simulink model "controllers"  (R2022a)
settings: Solver=FixedStepDiscrete  StartTime=0.0  StopTime=30  FixedStep=1  RelTol=1e-3  EnableMultiTasking=on
settings Model: ExtModeTrigDuration=2  Creator=Amin  LastModifiedBy=Parsa Noori
settings SolverCC: AlgebraicLoopSolver=TrustRegion
settings OptimizationCC: DefaultParameterBehavior=Inlined  UseDivisionForNetSlopeComputation=on  GainParamInheritBuiltInType=on  UseFloatMulNetSlope=on  InlineInvariantSignals=on  PassReuseOutputArgsAs=Individual arguments  ZeroExternalMemoryAtStartup=off  ZeroInternalMemoryAtStartup=off  NoFixptDivByZeroProtection=on  EfficientFloat2IntCast=on  LifeSpan=1  MaxStackSize=64  OptimizeBlockOrder=speed  DifferentSizesBufferReuse=on  EfficientTunableParamExpr=on
settings DebuggingCC: ParameterTunabilityLossMsg=error  UnconnectedInputMsg=warning  UnconnectedOutputMsg=warning  UnconnectedLineMsg=warning  SFMachineParentedDataDiag=warning
settings HardwareCC: ProdBitPerInt=16  ProdBitPerPointer=16  ProdBitPerSizeT=16  ProdBitPerPtrDiffT=16  ProdLargestAtomicFloat=None  ProdWordSize=8  ProdLongLongMode=on  ProdHWDeviceType=Atmel->AVR
settings SFSimCC: MATLABDynamicMemAlloc=off
settings RTWCC: SystemTargetFile=ert.tlc  HardwareBoard=Arduino Mega 2560  GenCodeOnly=on  TemplateMakefile=ert_default_tmf  Toolchain=Arduino AVR  BuildConfiguration=Faster Runs
settings CodeAppCC: ForceParamTrailComments=on  IgnoreCustomStorageClasses=off  OperatorAnnotations=on  SimulinkDataObjDesc=on  SFDataObjDesc=on  CustomSymbolStrGlobalVar=rt$N$M  CustomSymbolStrType=$N$M  CustomSymbolStrFcn=$N$M$F  CustomSymbolStrMacro=$N$M  InsertBlockDesc=on
settings ERTTargetCC: IncludeMdlTerminateFcn=off  CombineSignalStateStructs=on  SupportAbsoluteTime=off  PurelyIntegerCode=on  SupportComplex=off  SupportNonInlinedSFcns=on  ExtModeTransport=3  ExtModeStaticAlloc=on  ExtModeStaticAllocSize=2048  ExtModeMexFile=ext_xcp  ExtModeIntrfLevel=Level2 - Open  InlinedParameterPlacement=NonHierarchical  ERTFilePackagingFormat=CompactWithDataFile  IndentSize=4

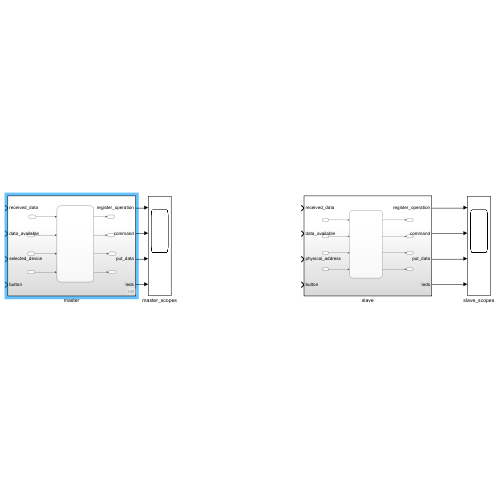
[thumbnail: Simulink's stored preview of the top-level diagram]
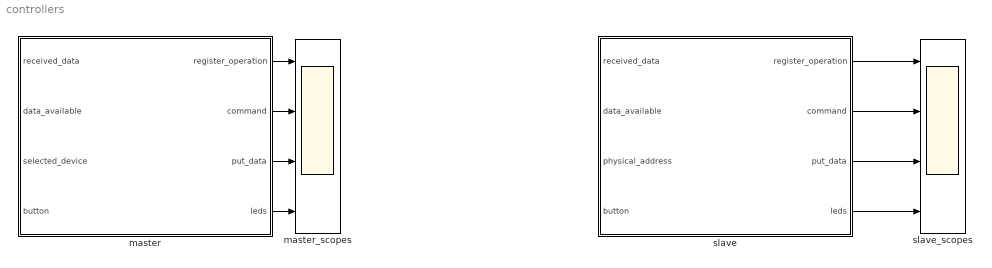
== system controllers ==
  master : Subsystem
  master_scopes : Scope  NumInputPorts=4
  slave : Subsystem
  slave_scopes : Scope  NumInputPorts=4
  wires:
  master/1(register_operation) -> master_scopes/1
  master/2(command) -> master_scopes/2
  master/3(put_data) -> master_scopes/3
  master/4(leds) -> master_scopes/4
  slave/1(register_operation) -> slave_scopes/1
  slave/2(command) -> slave_scopes/2
  slave/3(put_data) -> slave_scopes/3
  slave/4(leds) -> slave_scopes/4

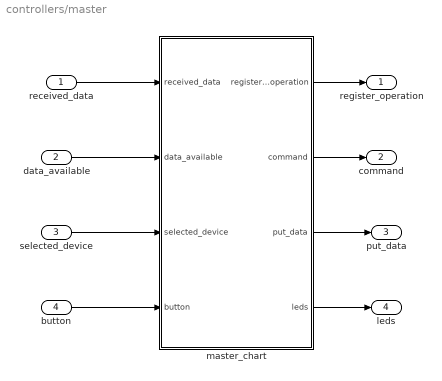
== system controllers/master ==
  received_data : Inport
  data_available : Inport  Port=2
  selected_device : Inport  Port=3
  button : Inport  Port=4
  master_chart : Stateflow chart  TreatAsAtomicUnit=on
      settings: PortSchema="{\"entries\":[{\"content\":{\"sides\":[{\"content\":{\"connectorIds\":[\"In1\",\"In2\",\"In3\",\"In4\"]},\"type\":\"ConnectorPlacement.EquallySpacedRectSide\",\"uuid\":\"138602be-6c58-4e8c-ba48-a14eddddc67c\"},{\"content\":{\"connectorIds\":[\"Out2\",\"Out1\",\"Out3\",\"Out4\"],\"side\":\"RIGHT\"},\"type\":\"ConnectorPlacement.EquallySpacedRectSide\",\"uuid\":\"5ecf324f-f194-43dd-983a-d068392304a8\"},{\"content\":{\"connectorIds\":[],\"side\":\"TOP\"},\"type\":\"ConnectorPlacement.EquallySpacedRectSide\",\"uuid\":\"4d10d79f-a1db-44f1-98c5-6d0be9e5b6d6\"}]},\"type\":\"ConnectorPlacement.EquallySpacedConnector\",\"uuid\":\"447fba48-e554-4a4b-a9f0-a545df5fe3d2\"}],\"packageUris\":[\"http://schema.mathworks.com/mf0/Connector/R2020b\"],\"version\":\"1.0\"}"
  register_operation : Outport
  command : Outport  Port=2
  put_data : Outport  Port=3  OutDataTypeStr=uint8
  leds : Outport  Port=4
  wires:
  received_data/1 -> master_chart/1(received_data)
  master_chart/1(command) -> command/1
  data_available/1 -> master_chart/2(data_available)
  master_chart/2(register_operation) -> register_operation/1
  master_chart/3(put_data) -> put_data/1
  selected_device/1 -> master_chart/3(selected_device)
  button/1 -> master_chart/4(button)
  master_chart/4(leds) -> leds/1

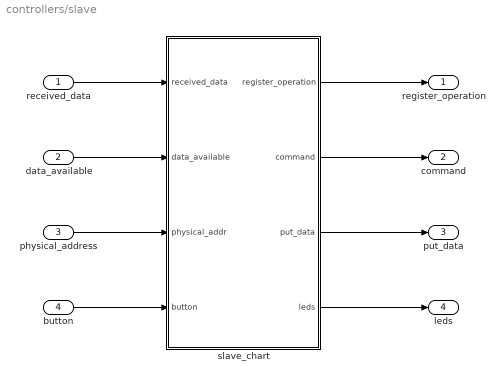
== system controllers/slave ==
  received_data : Inport
  data_available : Inport  Port=2
  physical_address : Inport  Port=3
  button : Inport  Port=4
  slave_chart : Stateflow chart  TreatAsAtomicUnit=on
      settings: PortSchema="{\"entries\":[{\"content\":{\"sides\":[{\"content\":{\"connectorIds\":[\"In1\",\"In2\",\"In3\",\"In4\"]},\"type\":\"ConnectorPlacement.EquallySpacedRectSide\",\"uuid\":\"138602be-6c58-4e8c-ba48-a14eddddc67c\"},{\"content\":{\"connectorIds\":[\"Out2\",\"Out1\",\"Out3\",\"Out4\"],\"side\":\"RIGHT\"},\"type\":\"ConnectorPlacement.EquallySpacedRectSide\",\"uuid\":\"5ecf324f-f194-43dd-983a-d068392304a8\"},{\"content\":{\"connectorIds\":[],\"side\":\"TOP\"},\"type\":\"ConnectorPlacement.EquallySpacedRectSide\",\"uuid\":\"4d10d79f-a1db-44f1-98c5-6d0be9e5b6d6\"}]},\"type\":\"ConnectorPlacement.EquallySpacedConnector\",\"uuid\":\"447fba48-e554-4a4b-a9f0-a545df5fe3d2\"}],\"packageUris\":[\"http://schema.mathworks.com/mf0/Connector/R2020b\"],\"version\":\"1.0\"}"
  register_operation : Outport
  command : Outport  Port=2
  put_data : Outport  Port=3  OutDataTypeStr=uint8
  leds : Outport  Port=4  OutDataTypeStr=uint8
  wires:
  received_data/1 -> slave_chart/1(received_data)
  slave_chart/1(command) -> command/1
  data_available/1 -> slave_chart/2(data_available)
  slave_chart/2(register_operation) -> register_operation/1
  slave_chart/3(put_data) -> put_data/1
  physical_address/1 -> slave_chart/3(physical_addr)
  slave_chart/4(leds) -> leds/1
  button/1 -> slave_chart/4(button)

== stateflow chart controllers/slave/slave_chart ==
  settings: updateMethod=DISCRETE  sampleTime=1
  state update_leds
  state wait_bus_idle
    during:
    idle_clocks = idle_clocks + 1;
  state bus_idle
    during:
    button_old = button
  state startup
  state wait_for_master
  state read_register_address
  state put_data
  state read_data
  state process_data
    entry:
    during:
    exit:
  state output  = combine_bits(bits) [function]
    (default) -> (junction 351)
    (junction 351) -> (junction 352) : {i = 0; output = 0}
    (junction 352) -> (junction 356) [order 1] : [i < sizeof(bits)]
    (junction 344) -> (junction 352) : {i = i + 1;}
    (junction 356) -> (junction 344) : {output |= bits[i] << i;}
    (junction 352) -> (junction 346) [order 2]
  state result  = button_pressed(old_state, current_state) [function]
    (default) -> (junction 336)
    (junction 336) -> (junction 334) : {result = 0}
    (junction 334) -> (junction 333) [order 1] : [result < sizeof(old_state)]
    (junction 333) -> (junction 334) [order 2] : {result = result + 1}
    (junction 333) -> (junction 331) [order 1] : [old_state[result] == 0 && current_state[result] == 1]
    (junction 334) -> (junction 331) [order 2]
  state results  = extract_bits(data) [function]
    (default) -> (junction 363)
    (junction 363) -> (junction 365) : {i = 0;}
    (junction 365) -> (junction 368) [order 1] : [i < sizeof(results)]
    (junction 366) -> (junction 365) : {i = i + 1;}
    (junction 368) -> (junction 366) : {results[i] = data & 0x1;
        | data = data >> 1;}
    (junction 365) -> (junction 364) [order 2]
  update_leds -> wait_bus_idle [order 3] : [from_wait_bus == true]{register_operation = 1;
      | command = 3;
      | button_old = button
      | idle_clocks = 0;}
  update_leds -> update_leds [order 1] : [button_pressed(button_old, button) != sizeof(button)]
  bus_idle -> wait_bus_idle [order 2] : [data_available == true && received_data != physical_addr]{register_operation = 1;
      | command = 3;
      | button_old = button
      | idle_clocks = 0;}
  wait_bus_idle -> update_leds [order 2] : [button_pressed(button_old, button) != sizeof(button)]{from_wait_bus = true;
      | command = 0;
      |
      | leds = leds ^ (button ^ button_old);
      | button_old = button;
      | }
  update_leds -> bus_idle [order 2] : [from_wait_bus == false]{register_operation = 1;
      | command = 2;}
  bus_idle -> update_leds [order 3] : [button_pressed(button_old, button) != sizeof(button)]{from_wait_bus = false;
      | command = 0;
      |
      | leds = leds ^ (button ^ button_old);
      | button_old = button;}
  wait_bus_idle -> bus_idle [order 1] : [idle_clocks >= 3]{register_operation = 1;
      | command = 2;}
  wait_bus_idle -> wait_bus_idle [order 3] : [data_available == true]{idle_clocks = 0}
  (default) -> startup : []{
      | command = 0;
      | leds = 0;
      | button_old = 0;}
  startup -> bus_idle : [true]{register_operation = 1;
      | command = 2;}
  read_register_address -> wait_for_master : [data_available == true]{
      | command = 0;}
  bus_idle -> read_register_address [order 1] : [data_available == true && received_data == physical_addr]{
      | register_operation = 1;
      | command = 2;}
  wait_for_master -> put_data [order 2] : [received_data == 128]{register_operation = 0;
      | command = 1;
      | put_data = combine_bits(leds)}
  wait_for_master -> read_data [order 1] : [received_data == 0]{
      | register_operation = 1;
      | command = 2;}
  (junction 107) -> bus_idle
  put_data -> (junction 107) : [true]{register_operation = 1;
      | command = 2;}
  read_data -> process_data : [data_available == true]{command = 0;
      |
      | leds =extract_bits(received_data);}
  process_data -> (junction 107) : [true]{register_operation = 1;
      | command = 2;}
  data: bits function_input uint8 size=[1 8]; output function_output uint8; i temporary uint8; old_state function_input uint8 size=[1 8]; current_state function_input uint8 size=[1 8]; result function_output uint8; data function_input uint8; results function_output uint8 size=[1 8]; i temporary uint8; received_data input uint8; command output uint8; data_available input boolean; register_operation output uint8; put_data output uint8; idle_clocks local uint8; physical_addr input uint8; button_old local uint8 size=[1 8]; leds output uint8 size=[1 8]; button input uint8 size=[1 8]; from_wait_bus local boolean

== stateflow chart controllers/master/master_chart ==
  settings: updateMethod=DISCRETE  sampleTime=1
  state bus_idle
  state retrieve_leds
  state update_leds
  state wait_bus_idle
    during:
    idle_clocks = idle_clocks + 1;
  state startup
  state send_physical_address
  state send_register_address
  state read_data
  state process_data
  state put_data
  state output  = combine_bits(bits) [function]
    (default) -> (junction 267)
    (junction 267) -> (junction 269) : {i = 0; output = 0}
    (junction 269) -> (junction 272) [order 1] : [i < sizeof(bits)]
    (junction 270) -> (junction 269) : {i = i + 1;}
    (junction 272) -> (junction 270) : {output |= bits[i] << i;}
    (junction 269) -> (junction 268) [order 2]
  state results  = extract_bits(data) [function]
    (default) -> (junction 258)
    (junction 258) -> (junction 253) : {i = 0;}
    (junction 253) -> (junction 261) [order 1] : [i < sizeof(results)]
    (junction 259) -> (junction 253) : {i = i + 1;}
    (junction 261) -> (junction 259) : {results[i] = data & 0x1;
        | data = data >> 1;}
    (junction 253) -> (junction 260) [order 2]
  state result  = button_pressed(old_state, current_state) [function]
    (default) -> (junction 180)
    (junction 180) -> (junction 173) : {result = 0}
    (junction 173) -> (junction 177) [order 1] : [result < sizeof(old_state)]
    (junction 177) -> (junction 173) [order 2] : {result = result + 1}
    (junction 177) -> (junction 175) [order 1] : [old_state[result] == 0 && current_state[result] == 1]
    (junction 173) -> (junction 175) [order 2]
  bus_idle -> retrieve_leds [order 1] : [retrieve_timeout == 0 | last_selected_device != selected_device]{command = 0;
      | phy_addr = uint8(selected_device);
      | reg_addr = (1 << 7) | 0;}
  wait_bus_idle -> bus_idle : [idle_clocks >= 5]{retrieve_timeout = 50;
      | command = 0;
      | button_old = button;
      | last_selected_device = selected_device;}
  bus_idle -> update_leds [order 2] : [button_pressed(button_old, button) != sizeof(button)]{command = 0;
      | leds = leds ^ (button ^ button_old);
      | button_old = button;
      | phy_addr = uint8(selected_device);
      | reg_addr = 0;}
  bus_idle -> bus_idle [order 3] : [retrieve_timeout > 0]{retrieve_timeout--}
  retrieve_leds -> send_physical_address : [true]{register_operation = 0;
      | command = 1;
      | put_data = uint8(phy_addr);}
  update_leds -> send_physical_address : [true]{register_operation = 0;
      | command = 1;
      | put_data = uint8(phy_addr);}
  (default) -> startup : []{command = 0;
      | phy_addr = uint8(selected_device);
      | reg_addr = 128;
      | leds = 0;
      | button_old = 0;}
  startup -> send_physical_address : [true] {register_operation = 0;
      | command = 1;
      | put_data = uint8(phy_addr);}
  send_physical_address -> send_register_address : [true]{register_operation = 0;
      | command = 1;
      | put_data = reg_addr;}
  process_data -> wait_bus_idle : [true]{command = 0;
      | idle_clocks = 0;}
  send_register_address -> read_data [order 2] : [reg_addr == 128]{register_operation = 1;
      | command = 2;}
  read_data -> process_data : [data_available == true]{command = 0;
      | leds = extract_bits(received_data)
      | }
  send_register_address -> put_data [order 1] : [reg_addr == 0]{register_operation = 0;
      | command = 1;
      | put_data = combine_bits(leds);}
  put_data -> wait_bus_idle : [true]{command = 0;
      | idle_clocks = 0;}
  data: bits function_input uint8 size=[1 8]; output function_output uint8; i temporary uint8; data function_input uint8; results function_output uint8 size=[1 8]; i temporary uint8; old_state function_input uint8 size=[1 8]; current_state function_input uint8 size=[1 8]; result function_output uint8; received_data input uint8; command output uint8; data_available input boolean; register_operation output uint8; put_data output uint8; idle_clocks local uint8; phy_addr local uint8; reg_addr local uint8; selected_device input uint8; leds output uint8 size=[1 8]; retrieve_timeout local uint8; button input uint8 size=[1 8]; button_old local uint8 size=[1 8]; last_selected_device local uint8
